simulink model "baloncuk_rov"  (R2024b)
settings: Solver=FixedStepDiscrete  StartTime=0.0  StopTime=inf  FixedStep=1e-3  RelTol=1e-3
model workspace (MAT data in the model file):
  ROTATE_CCW = 2
  ROTATE_CW = 1
  ROTATE_NONE = 0
libraries: simulink x19, utility x11, stm32f4xxblockslib x8, embeddedblockslib x2, stm32blockslib x2, dspstat3 x1
settings Model: STM32="{\"DigitalPortWrite\":[{\"ID\":\"untitled:3\"},{\"ID\":\"bldc_test:55\"},{\"ID\":\"baloncuk_rov:721\"},{\"ID\":\"baloncuk_rov:1493\"}],\"PWMOutput\":[{\"ID\":\"bldc_test:26\"},{\"ID\":\"bldc_test:37\"},{\"ID\":\"bldc_test:40\"},{\"ID\":\"bldc_test:45\"},{\"ID\":\"bldc_test:29\"},{\"ID\":\"bldc_test:74\"},{\"ID\":\"bldc_test:75\"},{\"ID\":\"bldc_test:76\"},{\"ID\":\"bldc_test:77\"},{\"ID\":\"baloncuk_rov:110\"},{\"ID\":\"baloncuk_rov:144\"},{\"ID\":\"baloncuk_rov:152\"},{\"ID\":\"baloncuk_rov:1586\"},{\"ID\":\"baloncuk_rov:1592\"}],\"TcpSend\":{\"ID\":\"bldc_test:62\"},\"TcpReceive\":{\"ID\":\"bldc_test:100\"},\"UdpReceive\":{\"ID\":\"baloncuk_rov:734\"},\"AnalogInput\":{\"ID\":\"baloncuk_rov:617\"},\"UdpSend\":{\"ID\":\"baloncuk_rov:1467\"}}"  SnapshotInterval=1000  Creator=loq  LastModifiedBy=loq
settings SolverCC: PositivePriorityOrder=on
settings OptimizationCC: UseDivisionForNetSlopeComputation=on  GainParamInheritBuiltInType=on  UseFloatMulNetSlope=on  UseSpecifiedMinMax=on  PassReuseOutputArgsAs=Individual arguments  ZeroExternalMemoryAtStartup=off  ZeroInternalMemoryAtStartup=off  NoFixptDivByZeroProtection=on  EfficientFloat2IntCast=on  LifeSpan=1  MaxStackSize=512  OptimizeBlockOrder=speed  DifferentSizesBufferReuse=on  EfficientTunableParamExpr=on
settings DebuggingCC: SignalInfNanChecking=warning  IntegerOverflowMsg=error  ParameterTunabilityLossMsg=error  AssertControl=DisableAll  SFUndirectedBroadcastEventsDiag=error
settings HardwareCC: ProdBitPerPointer=32  ProdBitPerSizeT=32  ProdBitPerPtrDiffT=32  ProdLargestAtomicInteger=Long  ProdLargestAtomicFloat=Double  ProdWordSize=32  ProdLongLongMode=on  ProdHWDeviceType=ARM Compatible->ARM Cortex-M
settings SFSimCC: SimCustomHeaderCode="#include \"bno08x_rvc_usart2_hal.h\""  SimUserSources=bno08x_rvc_usart2_hal.c  SimUserIncludeDirs=.\Core\Inc .\Core\Src .\baloncuk_rov_ert_rtw .\Drivers\CMSIS\Include .\Drivers\CMSIS\Device\ST\STM32F4xx\Include .\Drivers\STM32F4xx_HAL_Driver\Inc .\Drivers\STM32F4xx_HAL_Driver\Src  SimUserDefines=STM32F439xx  CompileTimeRecursionLimit=0  EnableRuntimeRecursion=off  MATLABDynamicMemAlloc=off
settings RTWCC: Description=Embedded Coder  SystemTargetFile=ert.tlc  HardwareBoard=STM32F4xx Based  TLCOptions="-aInlineSetEventsForThisBaseRateFcn=TLC_FALSE -aSuppressMultiTaskScheduler=TLC_FALSE   -aRateBasedStepFcn=1"  TemplateMakefile=ert_default_tmf  RTWUseSimCustomCode=on  CustomHeaderCode="#include \"bno08x_rvc_usart2_hal.h\""  CustomInclude=.\Core\Inc .\Core\Src .\baloncuk_rov_ert_rtw .\Drivers\CMSIS\Include .\Drivers\CMSIS\Device\ST\STM32F4xx\Include .\Drivers\STM32F4xx_HAL_Driver\Inc .\Drivers\STM32F4xx_HAL_Driver\Src  CustomSource=bno08x_rvc_usart2_hal.c  CustomDefine=STM32F439xx  Toolchain=GNU Tools for ARM Embedded Processors  BuildConfiguration=Faster Runs
settings CodeAppCC: ForceParamTrailComments=on  IgnoreCustomStorageClasses=off  OperatorAnnotations=on  SimulinkDataObjDesc=on  SFDataObjDesc=on  MATLABFcnDesc=on  InsertBlockDesc=on
settings ERTTargetCC: TargetLangStandard=C99 (ISO)  CodeReplacementLibrary=ARM Cortex-M  UtilityFuncGeneration=Shared location  CombineSignalStateStructs=on  SuppressErrorStatus=on  SupportNonFinite=off  ParenthesesLevel=Standards  CastingMode=Standards  GenerateSharedConstants=off  ExtModeTransport=3  ExtModeStaticAlloc=on  ExtModeStaticAllocSize=2048  ExtModeMexFile=ext_xcp  ExtModeIntrfLevel=Level2 - Open  InlinedParameterPlacement=Hierarchical  EnableSignedLeftShifts=off  EnableSignedRightShifts=off

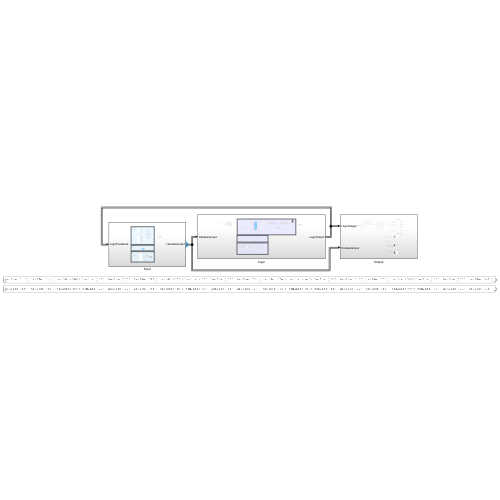
[thumbnail: Simulink's stored preview of the top-level diagram]
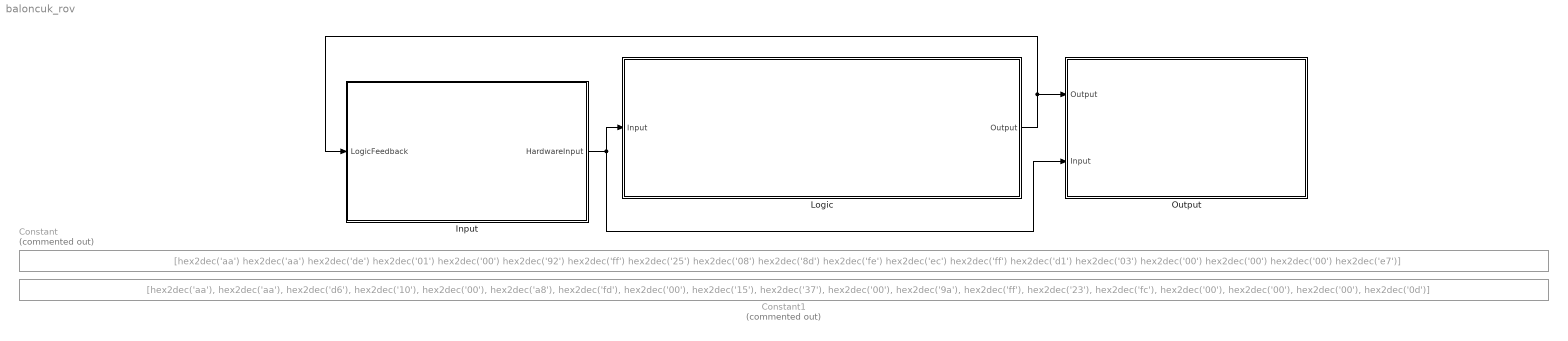
== system baloncuk_rov ==
  Constant : Constant  Commented=on  Value=[hex2dec('aa') hex2dec('aa') hex2dec('de') hex2dec('01') hex2dec('00') hex2dec('92') hex2dec('ff') hex2dec('25') hex2dec('08') hex2dec('8d') hex2dec('fe') hex2dec('ec') hex2dec('ff') hex2dec('d1') hex2dec('03') hex2dec('00') hex2dec('00') hex2dec('00') hex2dec('e7')]  OutDataTypeStr=uint8
  Constant1 : Constant  Commented=on  Value=[hex2dec('aa'), hex2dec('aa'), hex2dec('d6'), hex2dec('10'), hex2dec('00'), hex2dec('a8'), hex2dec('fd'), hex2dec('00'), hex2dec('15'), hex2dec('37'), hex2dec('00'), hex2dec('9a'), hex2dec('ff'), hex2dec('23'), hex2dec('fc'), hex2dec('00'), hex2dec('00'), hex2dec('00'), hex2dec('0d')]  OutDataTypeStr=uint8
  Input : Subsystem
  Logic : Subsystem
  Output : Subsystem
  wires:
  Input/1(HardwareInput) -> Logic/1(Input), Output/2(Input)
  Logic/1(Output) -> Input/1(LogicFeedback), Output/1(Output)

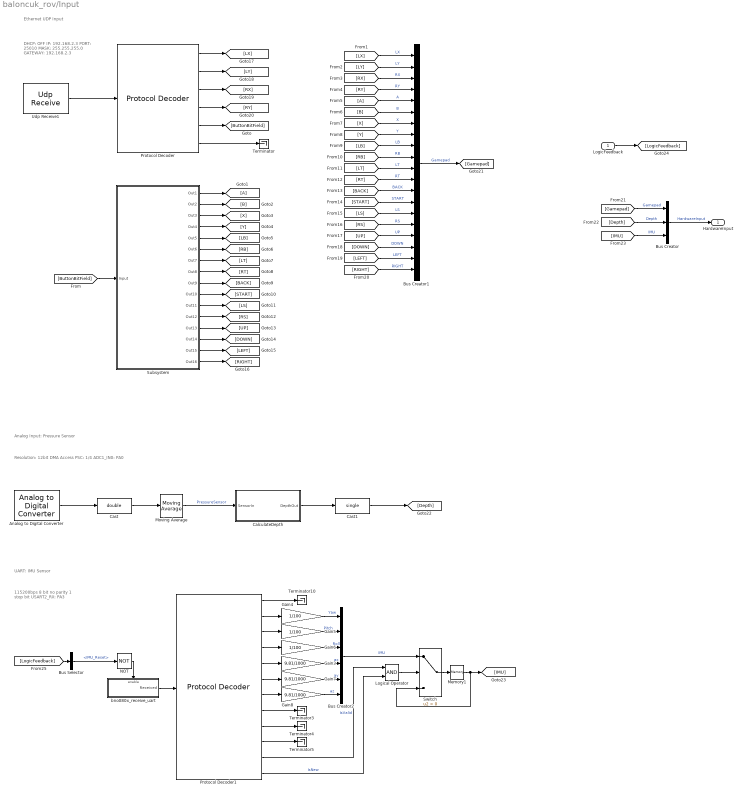
== system baloncuk_rov/Input ==
  note: Ethernet UDP Input
  note: DHCP: OFF
      | IP: 192.168.2.3
      | PORT: 25010
      | MASK: 255.255.255.0
      | GATEWAY: 192.168.2.3
  note: Analog Input: Pressure Sensor
  note: Resolution: 12bit
      | DMA Access
      | PSC: 1/4
      | ADC1_IN0: PA0
  note: UART: IMU Sensor
  note: 115200bps
      | 8 bit
      | no parity
      | 1 stop bit
      |
      | USART2_RX: PA3
  LogicFeedback : Inport
  Analog to Digital Converter : stm32f4xxblockslib/Analog to Digital Converter  ADCModule=ADC1  ConversionGroup=Regular  TriggerMode=Trigger and read  NumberOfConversions=1  EnableBufferConv=off  BufferLength=1  OutputStatus=off  SampleTime=-1  EnableSimPort=off  hoistedMaskSrc=ECSoC/ECSimCodegen/Analog to Digital Converter
  Bus Creator : BusCreator  Inputs=3
  Bus Creator1 : BusCreator  Inputs=20
  Bus Creator2 : BusCreator  Inputs=6
  Bus Selector : BusSelector  OutputSignals=IMU_Bus.IMU_Reset
  CalculateDepth : Subsystem
  Cast : DataTypeConversion  OutDataTypeStr=double  SaturateOnIntegerOverflow=off  RndMeth=Floor
  Cast1 : DataTypeConversion  OutDataTypeStr=single  SaturateOnIntegerOverflow=off  RndMeth=Floor
  From5 : From
  Gain3 : Gain  Gain=9.81/1000  OutDataTypeStr=single
  Gain4 : Gain  Gain=1/100  OutDataTypeStr=single
  Gain5 : Gain  Gain=1/100  OutDataTypeStr=single
  Gain6 : Gain  Gain=1/100  OutDataTypeStr=single
  Gain7 : Gain  Gain=9.81/1000  OutDataTypeStr=single
  Gain8 : Gain  Gain=9.81/1000  OutDataTypeStr=single
  Goto1 : Goto
  Logical Operator : Logic  AllPortsSameDT=off  OutDataTypeStr=boolean
  Memory1 : Memory
  Moving Average : dspstat3/Moving Average  Method=Sliding window  ForgettingFactorPort=off  SpecifyWindowLength=on  WindowLength=1/0.005  OverlapLength=199  AllowArbitraryInputLength=off  ForgettingFactor=0.9  SimulateUsing=Interpreted execution
  NOT : Logic  Operator=NOT  IconShape=distinctive  AllPortsSameDT=off  OutDataTypeStr=boolean
  Protocol Decoder : embeddedblockslib/Protocol Decoder  IsParseCSV=off  Header=[13]  FieldTable={ 'LX', '1', 'int8', 'Little endian'; 'LY', '1', 'int8', 'Little endian'; 'RX', '1', 'int8', 'Little endian'; 'RY', '1', 'int8', 'Little endian'; 'ButtonBitField', '1', 'uint16', 'Little endian' }  IsVariableSizeLastField=off  MaxVariableSizeFieldLength=[]  IsChecksumRequired=off  ChecksumAlgorithm=XOR of bytes  ChecksumSize=[]  TerminatorOption=Custom terminator  CustomTerminatorVal=[10]  IsInputLengthAvailable=off
      settings: LibrarySourceBlock=stmutilitieslib/Protocol Decoder
  Protocol Decoder1 : embeddedblockslib/Protocol Decoder  IsParseCSV=off  Header=[hex2dec('aa') hex2dec('aa')]  FieldTable={ 'Index', '1', 'uint8', 'Little endian'; 'Yaw', '1', 'int16', 'Little endian'; 'Pitch', '1', 'int16', 'Little endian'; 'Roll', '1', 'int16', 'Little endian'; 'X_Accel', '1', 'int16', 'Little endian'; 'Y_Accel', '1', 'int16', 'Little endian'; 'Z_Accel', '1', 'int16', 'Little endian'; 'Res_0', '1', 'uint8', 'Little endian'; 'Res_1', '1', 'uint8', 'Little endian'; 'Res_2', '1', 'uint8', 'Little endian' }  IsVariableSizeLastField=off  MaxVariableSizeFieldLength=[]  IsChecksumRequired=on  ChecksumAlgorithm=Custom algorithm  ChecksumSize=1  ChecksumFilepath=C:\Users\loq\Documents\MATLAB\baloncuk_rov\bno08x_checksum.m  TerminatorOption=<none>  CustomTerminatorVal=[10]  IsInputLengthAvailable=off
      settings: LibrarySourceBlock=stmutilitieslib/Protocol Decoder
  Subsystem : Subsystem
  Switch : Switch  Criteria=u2 > Threshold  SaturateOnIntegerOverflow=off  InputSameDT=off
  Terminator{,3..5,10} (5 alike) : Terminator
  Udp Receive1 : stm32blockslib/Udp Receive  Direction=Receive  RemoteIPAddress=192.168.2.2  LocalPort=25010  RemoteIPPort=25002  ByteOrder=LittleEndian  BlockingMode=off  BlockTimeout=0.1  DataType=uint8  DataLength=8  OutputStatus=off  SampleTime=-1
      settings: LibrarySourceBlock=stm32f4xxblockslib/Udp Receive
  bno080x_receive_uart : Subsystem  TreatAsAtomicUnit=on
  HardwareInput : Outport
  wires:
  Subsystem/15(Out15) -> [LEFT]
  [ButtonBitField] -> Subsystem/1(Input)
  Subsystem/12(Out12) -> [RS]
  Subsystem/14(Out14) -> [DOWN]
  Subsystem/1(Out1) -> Goto1/1
  Protocol Decoder/6 -> Terminator/1
  Protocol Decoder/2 -> [LY]
  Subsystem/3(Out3) -> [X]
  Protocol Decoder/4 -> [RY]
  Subsystem/10(Out10) -> [START]
  Subsystem/11(Out11) -> [LS]
  Subsystem/7(Out7) -> [LT]
  Protocol Decoder/5 -> [ButtonBitField]
  Subsystem/6(Out6) -> [RB]
  Subsystem/8(Out8) -> [RT]
  Udp Receive1/1 -> Protocol Decoder/1
  Protocol Decoder/1 -> [LX]
  Subsystem/5(Out5) -> [LB]
  Protocol Decoder/3 -> [RX]
  Subsystem/16(Out16) -> [RIGHT]
  Subsystem/2(Out2) -> [B]
  Subsystem/9(Out9) -> [BACK]
  Subsystem/4(Out4) -> [Y]
  Subsystem/13(Out13) -> [UP]
  [LX] -> Bus Creator1/1  "LX"
  [LY] -> Bus Creator1/2  "LY"
  [RX] -> Bus Creator1/3  "RX"
  [RY] -> Bus Creator1/4  "RY"
  From5/1 -> Bus Creator1/5  "A"
  [B] -> Bus Creator1/6  "B"
  [X] -> Bus Creator1/7  "X"
  [Y] -> Bus Creator1/8  "Y"
  [LB] -> Bus Creator1/9  "LB"
  [RB] -> Bus Creator1/10  "RB"
  [LT] -> Bus Creator1/11  "LT"
  [RT] -> Bus Creator1/12  "RT"
  [BACK] -> Bus Creator1/13  "BACK"
  [START] -> Bus Creator1/14  "START"
  [LS] -> Bus Creator1/15  "LS"
  [RS] -> Bus Creator1/16  "RS"
  [UP] -> Bus Creator1/17  "UP"
  [DOWN] -> Bus Creator1/18  "DOWN"
  [LEFT] -> Bus Creator1/19  "LEFT"
  [RIGHT] -> Bus Creator1/20  "RIGHT"
  Bus Creator/1 -> HardwareInput/1  "HardwareInput"
  Bus Creator1/1 -> [Gamepad]  "Gamepad"
  [Gamepad] -> Bus Creator/1  "Gamepad"
  Cast/1 -> Moving Average/1
  Analog to Digital Converter/1 -> Cast/1
  Moving Average/1 -> CalculateDepth/1(SensorIn)  "PressureSensor"
  CalculateDepth/1(DepthOut) -> Cast1/1
  [Depth] -> Bus Creator/2  "Depth"
  [IMU] -> Bus Creator/3  "IMU"
  Gain3/1 -> Bus Creator2/4  "ax"
  Protocol Decoder1/6 -> Gain7/1
  Protocol Decoder1/5 -> Gain3/1
  Gain7/1 -> Bus Creator2/5  "ay"
  Bus Creator2/1 -> Switch/1  "IMU"
  Protocol Decoder1/1 -> Terminator10/1
  Gain6/1 -> Bus Creator2/3  "Roll"
  Protocol Decoder1/4 -> Gain6/1
  Protocol Decoder1/2 -> Gain4/1
  Gain4/1 -> Bus Creator2/1  "Yaw"
  Protocol Decoder1/9 -> Terminator4/1
  Gain8/1 -> Bus Creator2/6  "az"
  Protocol Decoder1/12 -> Logical Operator/2  "IsNew"
  Protocol Decoder1/7 -> Gain8/1
  Protocol Decoder1/11 -> Logical Operator/1  "IsValid"
  Protocol Decoder1/8 -> Terminator3/1
  Gain5/1 -> Bus Creator2/2  "Pitch"
  Protocol Decoder1/3 -> Gain5/1
  Protocol Decoder1/10 -> Terminator5/1
  Logical Operator/1 -> Switch/2
  Switch/1 -> Memory1/1
  Memory1/1 -> Switch/3, [IMU]
  bno080x_receive_uart/1(Received) -> Protocol Decoder1/1
  NOT/1 -> bno080x_receive_uart/Enable
  LogicFeedback/1 -> [LogicFeedback]
  [LogicFeedback] -> Bus Selector/1
  Bus Selector/1 -> NOT/1  "<IMU_Reset>"
  Cast1/1 -> [Depth]

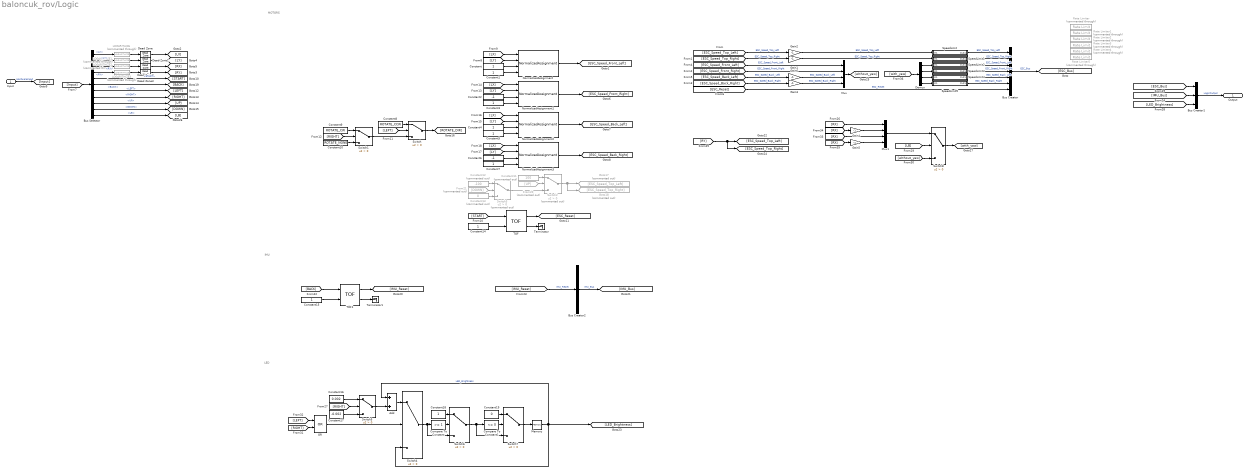
== system baloncuk_rov/Logic ==
  note: LED
  note: MOTORS
  note: IMU
  Input : Inport
  Add : Sum
  Bus Creator : BusCreator  Inputs=7
  Bus Creator1 : BusCreator  Inputs=3
  Bus Creator2 : BusCreator  Inputs=1
  Bus Selector : BusSelector  OutputSignals=Gamepad.LX,Gamepad.LY,Gamepad.RX,Gamepad.RY,Gamepad.START,Gamepad.BACK,Gamepad.LEFT,Gamepad.RIGHT,Gamepad.UP,Gamepad.DOWN,Gamepad.LB
  Compare To Constant : simulink/Logic and Bit Operations/Compare To Constant  relop=>=  const=1  OutDataTypeStr=boolean
  Compare To Constant1 : simulink/Logic and Bit Operations/Compare To Constant  relop=<=  const=0  OutDataTypeStr=boolean
  Constant{,1,3..5,7} (6 alike) : Constant  OutDataTypeStr=int8
  Constant10 : Constant  Value=ROTATE_NONE
  Constant11 : Constant  Commented=on  Value=100  OutDataTypeStr=int8
  Constant12 : Constant  Commented=on  Value=-100  OutDataTypeStr=int8
  Constant13 : Constant  Commented=on  Value=0  OutDataTypeStr=int8
  Constant14 : Constant  OutDataTypeStr=single
  Constant15 : Constant  OutDataTypeStr=single
  Constant16 : Constant  Value=0.002
  Constant17 : Constant  Value=-0.002
  Constant18 : Constant
  Constant19 : Constant  Value=0
  Constant2 : Constant  Value=-1  OutDataTypeStr=int8
  Constant6 : Constant  Value=-1  OutDataTypeStr=int8
  Constant8 : Constant  Value=ROTATE_CCW
  Constant9 : Constant  Value=ROTATE_CW
  Dead Zone{,1..3} (4 alike) : DeadZone  LowerValue=-5  UpperValue=5
  Demux : Demux
  From20 : From  Commented=on  GotoTag=UP
  From21 : From  Commented=on  GotoTag=DOWN
  Gain{1..4,6} (5 alike) : Gain  Gain=-1  OutDataTypeStr=int8
  Gain5 : Gain  Gain=-1  ParamDataTypeStr=int8  OutDataTypeStr=int8
  Goto17 : Goto  Commented=on  GotoTag=ESC_Speed_Top_Left
  Goto18 : Goto  Commented=on  GotoTag=ESC_Speed_Top_Right
  LOGARITHIZE{,1..3} (4 alike) : utility/LOGARITHIZE  Commented=through  SystemSampleTime=-1  VariantActivationTime=update diagram  AllowFlexibleInterface=on  Latency=0  AutoFrameSizeCalculation=off
  Memory : Memory  InitialCondition=0.00  InheritSampleTime=on
  Mux : Mux
  Mux1 : Mux
  NormalizedAssignment{,1..3} (4 alike) : utility/NormalizedAssignment  SystemSampleTime=-1  VariantActivationTime=update diagram  AllowFlexibleInterface=on  Latency=0  AutoFrameSizeCalculation=off
  OR : Logic  Operator=OR  AllPortsSameDT=off  OutDataTypeStr=boolean
  Rate Limiter{,1..5} (6 alike) : RateLimiter  Commented=through  RisingSlewLimit=10  FallingSlewLimit=-10  SampleTimeMode=inherited
  SpeedLimit : Subsystem
  SpeedLimit1 : Subsystem
  SpeedLimit2 : Subsystem
  SpeedLimit3 : Subsystem
  SpeedLimit4 : Subsystem
  SpeedLimit5 : Subsystem
  Switch{,1,4..8} (7 alike) : Switch  Criteria=u2 > Threshold  SaturateOnIntegerOverflow=off  InputSameDT=off
  Switch2 : Switch  Commented=on  Criteria=u2 > Threshold  SaturateOnIntegerOverflow=off  InputSameDT=off
  Switch3 : Switch  Commented=on  Criteria=u2 > Threshold  SaturateOnIntegerOverflow=off  InputSameDT=off
  TOF : utility/TOF  SystemSampleTime=-1  VariantActivationTime=update diagram  AllowFlexibleInterface=on  Latency=0  AutoFrameSizeCalculation=off
  TOF1 : utility/TOF  SystemSampleTime=-1  VariantActivationTime=update diagram  AllowFlexibleInterface=on  Latency=0  AutoFrameSizeCalculation=off
  Terminator : Terminator
  Terminator1 : Terminator
  Output : Outport
  wires:
  [ESC_Speed_Top_Left] -> Gain2/1  "ESC_Speed_Top_Left"
  [ESC_Speed_Top_Right] -> Gain1/1  "ESC_Speed_Top_Right"
  [ESC_Speed_Front_Right] -> Mux/2  "ESC_Speed_Front_Right"
  [ESC_Speed_Back_Left] -> Gain6/1  "ESC_Speed_Back_Left"
  [ESC_Speed_Front_Left] -> Mux/1  "ESC_Speed_Front_Left"
  [ESC_Reset] -> Bus Creator/7  "ESC_Reset"
  Bus Creator/1 -> [ESC_Bus]  "ESC_Bus"
  Input/1 -> [Input]  "HardwareInput"
  Bus Selector/1 -> LOGARITHIZE/1  "<LX>"
  Bus Selector/4 -> LOGARITHIZE3/1  "<RY>"
  Bus Selector/2 -> LOGARITHIZE1/1  "<LY>"
  Bus Selector/3 -> LOGARITHIZE2/1  "<RX>"
  NormalizedAssignment/1 -> [ESC_Speed_Front_Left]
  [LX] -> NormalizedAssignment/1
  [LY] -> NormalizedAssignment/2
  Constant/1 -> NormalizedAssignment/3
  Constant1/1 -> NormalizedAssignment/4
  Constant3/1 -> NormalizedAssignment1/4
  Constant2/1 -> NormalizedAssignment1/3
  [LY] -> NormalizedAssignment1/2
  [LX] -> NormalizedAssignment1/1
  NormalizedAssignment1/1 -> [ESC_Speed_Front_Right]
  NormalizedAssignment2/1 -> [ESC_Speed_Back_Left]
  [LX] -> NormalizedAssignment2/1
  [LY] -> NormalizedAssignment2/2
  Constant4/1 -> NormalizedAssignment2/3
  Constant5/1 -> NormalizedAssignment2/4
  Constant7/1 -> NormalizedAssignment3/4
  Constant6/1 -> NormalizedAssignment3/3
  [LX] -> NormalizedAssignment3/1
  NormalizedAssignment3/1 -> [ESC_Speed_Back_Right]
  [Input] -> Bus Selector/1
  Bus Selector/5 -> [START]  "<START>"
  Bus Selector/7 -> [LEFT]  "<LEFT>"
  Bus Selector/8 -> [RIGHT]  "<RIGHT>"
  Bus Selector/9 -> [UP]  "<UP>"
  Bus Selector/10 -> [DOWN]  "<DOWN>"
  [LEFT] -> Switch/2
  Constant8/1 -> Switch/1
  Constant9/1 -> Switch1/1
  [RIGHT] -> Switch1/2
  Switch1/1 -> Switch/3
  Switch/1 -> [ROTATE_DIR]
  Constant10/1 -> Switch1/3
  [ESC_Bus] -> Bus Creator1/1
  Bus Creator1/1 -> Output/1  "LogicOutput"
  Switch2/1 -> Goto18/1, Goto17/1
  From20/1 -> Switch2/2
  Constant11/1 -> Switch2/1
  Constant12/1 -> Switch3/1
  From21/1 -> Switch3/2
  Switch3/1 -> Switch2/3
  Constant13/1 -> Switch3/3
  [START] -> TOF/1
  TOF/1 -> [ESC_Reset]
  Constant14/1 -> TOF/2
  TOF/2 -> Terminator/1
  LOGARITHIZE/1 -> Dead Zone/1
  LOGARITHIZE1/1 -> Dead Zone1/1
  LOGARITHIZE2/1 -> Dead Zone2/1
  LOGARITHIZE3/1 -> Dead Zone3/1
  Bus Selector/6 -> [BACK]  "<BACK>"
  TOF1/2 -> Terminator1/1
  Constant15/1 -> TOF1/2
  TOF1/1 -> [IMU_Reset]
  [BACK] -> TOF1/1
  Bus Creator2/1 -> [IMU_Bus]  "IMU_Bus"
  [IMU_Reset] -> Bus Creator2/1  "IMU_Reset"
  [IMU_Bus] -> Bus Creator1/2
  [LED_Brightness] -> Bus Creator1/3
  Switch4/1 -> Switch6/3, Compare To Constant/1
  [LEFT] -> OR/1
  Switch7/1 -> Memory/1
  Constant17/1 -> Switch5/3
  [RIGHT] -> OR/2
  Constant16/1 -> Switch5/1
  Switch5/1 -> Add/2
  Memory/1 -> [LED_Brightness], Add/1, Switch4/3  "LED_Brightness"
  [RIGHT] -> Switch5/2
  OR/1 -> Switch4/2
  Constant18/1 -> Switch6/1
  Constant19/1 -> Switch7/1
  Compare To Constant1/1 -> Switch7/2
  Add/1 -> Switch4/1
  Switch6/1 -> Switch7/3, Compare To Constant1/1
  Compare To Constant/1 -> Switch6/2
  Gain1/1 -> SpeedLimit1/1(In1)  "ESC_Speed_Top_Right"
  [LY] -> NormalizedAssignment3/2
  Dead Zone/1 -> [LX]
  Dead Zone1/1 -> [LY]
  Dead Zone2/1 -> [RX]
  Dead Zone3/1 -> [RY]
  SpeedLimit/1(Out1) -> Bus Creator/1  "ESC_Speed_Top_Left"
  SpeedLimit1/1(Out1) -> Bus Creator/2  "ESC_Speed_Top_Right"
  SpeedLimit2/1(Out1) -> Bus Creator/3  "ESC_Speed_Front_Left"
  SpeedLimit3/1(Out1) -> Bus Creator/4  "ESC_Speed_Front_Right"
  SpeedLimit4/1(Out1) -> Bus Creator/5  "ESC_Speed_Back_Left"
  SpeedLimit5/1(Out1) -> Bus Creator/6  "ESC_Speed_Back_Right"
  [RY] -> [ESC_Speed_Top_Right], [ESC_Speed_Top_Left]
  [ESC_Speed_Back_Right] -> Gain3/1  "ESC_Speed_Back_Right"
  Mux/1 -> [without_yaw]
  Bus Selector/11 -> [LB]  "<LB>"
  [LB] -> Switch8/2
  [without_yaw] -> Switch8/3
  [RX] -> Mux1/1
  [RX] -> Mux1/3
  [RX] -> Gain4/1
  [RX] -> Gain5/1
  Gain4/1 -> Mux1/2
  Gain5/1 -> Mux1/4
  Mux1/1 -> Switch8/1
  Switch8/1 -> [with_yaw]
  [with_yaw] -> Demux/1
  Demux/1 -> SpeedLimit2/1(In1)
  Demux/2 -> SpeedLimit3/1(In1)
  Demux/3 -> SpeedLimit4/1(In1)
  Demux/4 -> SpeedLimit5/1(In1)
  Gain2/1 -> SpeedLimit/1(In1)  "ESC_Speed_Top_Left"
  Gain3/1 -> Mux/4  "ESC_Speed_Back_Right"
  Gain6/1 -> Mux/3  "ESC_Speed_Back_Left"

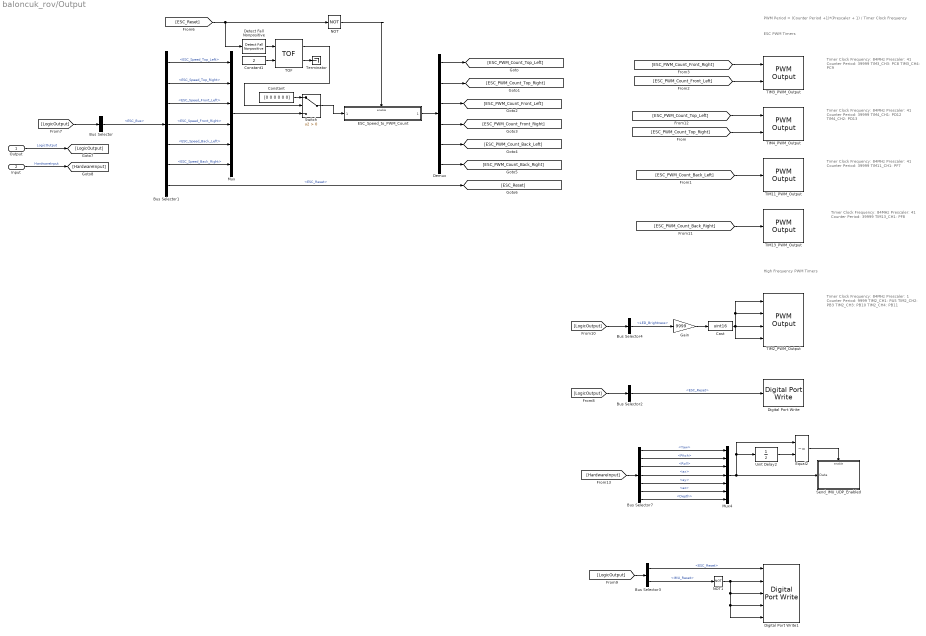
== system baloncuk_rov/Output ==
  note: PWM Period = (Counter Period +1)*(Prescaler + 1) / Timer Clock Frequency
  note: ESC PWM Timers
  note: Timer Clock Frequency: 84MHz
      | Prescaler: 41
      | Counter Period: 39999
      |
      | TIM3_CH3: PC8
      | TIM3_CH4: PC9
  note: High Frequency PWM Timers
  note: Timer Clock Frequency: 84MHz
      | Prescaler: 1
      | Counter Period: 9999
      |
      | TIM2_CH1: PA5
      | TIM2_CH2: PB3
      | TIM2_CH3: PB10
      | TIM2_CH4: PB11
  note: Timer Clock Frequency: 84MHz
      | Prescaler: 41
      | Counter Period: 39999
      |
      | TIM4_CH1: PD12
      | TIM4_CH2: PD13
  note: Timer Clock Frequency: 84MHz
      | Prescaler: 41
      | Counter Period: 39999
      |
      | TIM11_CH1: PF7
  note: Timer Clock Frequency: 84MHz
      | Prescaler: 41
      | Counter Period: 39999
      |
      | TIM13_CH1: PF8
  Output : Inport
  Input : Inport  Port=2
  Bus Selector : BusSelector  OutputSignals=ESC_Bus
  Bus Selector1 : BusSelector  OutputSignals=ESC_Speed_Top_Left,ESC_Speed_Top_Right,ESC_Speed_Front_Left,ESC_Speed_Front_Right,ESC_Speed_Back_Left,ESC_Speed_Back_Right,ESC_Reset
  Bus Selector2 : BusSelector  OutputSignals=ESC_Bus.ESC_Reset
  Bus Selector3 : BusSelector  OutputSignals=ESC_Bus.ESC_Reset,IMU_Bus.IMU_Reset
  Bus Selector4 : BusSelector  OutputSignals=LED_Brightness
  Bus Selector7 : BusSelector  OutputSignals=IMU.Yaw,IMU.Pitch,IMU.Roll,IMU.ax,IMU.ay,IMU.az,Depth
  Cast : DataTypeConversion  OutDataTypeStr=uint16  SaturateOnIntegerOverflow=off  RndMeth=Floor
  Constant : Constant  Value=[0 0 0 0 0 0]
  Constant1 : Constant  Value=2  OutDataTypeStr=single
  Demux : Demux  Outputs=6
  Detect Fall Nonpositive : simulink/Logic and Bit Operations/Detect Fall Nonpositive  vinit=0  OutDataTypeStr=boolean
  Digital Port Write : stm32f4xxblockslib/Digital Port Write  PortName=GPIOB  PinNumber=7  ReadOperation=off  IOAsArray=off  EnableSimPort=off  hoistedMaskSrc=ECSoC/ECSimCodegen/Digital Port Write
  Digital Port Write1 : stm32f4xxblockslib/Digital Port Write  PortName=GPIOE  PinNumber=[2 3 4 5 6]  ReadOperation=off  IOAsArray=off  EnableSimPort=off  hoistedMaskSrc=ECSoC/ECSimCodegen/Digital Port Write
  ESC_Speed_to_PWM_Count : Subsystem  ReferencedSubsystem=ESC_Speed_to_PWM_Count
  Equal2 : RelationalOperator  Operator=~=  OutDataTypeStr=boolean  RndMeth=Simplest  InputSameDT=off
  Gain : Gain  Gain=9999
  Mux : Mux  Inputs=6
  Mux4 : Mux  Inputs=7
  NOT : Logic  Operator=NOT  IconShape=distinctive  AllPortsSameDT=off  OutDataTypeStr=boolean
  NOT1 : Logic  Operator=NOT  IconShape=distinctive  AllPortsSameDT=off  OutDataTypeStr=boolean
  Send_IMU_UDP_Enabled : Subsystem  TreatAsAtomicUnit=on
  Switch : Switch  Criteria=u2 > Threshold  SaturateOnIntegerOverflow=off  InputSameDT=off
  TIM11_PWM_Output : stm32f4xxblockslib/PWM Output  TimerModule=TIM11  DutycycleUnits=Counts  EnableChannel1=on  EnableChannel2=on  EnableChannel3=on  EnableChannel4=on  EnableCounterInput=off  EnableMainOutputInput=off  EnableFrequencyInput=off  SetRCAfterCE=off  OutputDirection=off  OutputMainOutputEnableStatus=off  SampleTime=0.1  EnableSimPort=off  EnableUpdateEvent=off  EnableCaptureCompare1Event=off  EnableCaptureCompare2Event=off  EnableCaptureCompare3Event=off  EnableCaptureCompare4Event=off  EnableTriggerEvent=off  EnableBreakEvent=off  ProcessorFamily=STM32F4  hoistedMaskSrc=ECSoC/ECSimCodegen/PWM Output
  TIM13_PWM_Output : stm32f4xxblockslib/PWM Output  TimerModule=TIM13  DutycycleUnits=Counts  EnableChannel1=on  EnableChannel2=on  EnableChannel3=on  EnableChannel4=on  EnableCounterInput=off  EnableMainOutputInput=off  EnableFrequencyInput=off  SetRCAfterCE=off  OutputDirection=off  OutputMainOutputEnableStatus=off  SampleTime=0.1  EnableSimPort=off  EnableUpdateEvent=off  EnableCaptureCompare1Event=off  EnableCaptureCompare2Event=off  EnableCaptureCompare3Event=off  EnableCaptureCompare4Event=off  EnableTriggerEvent=off  EnableBreakEvent=off  ProcessorFamily=STM32F4  hoistedMaskSrc=ECSoC/ECSimCodegen/PWM Output
  TIM2_PWM_Output : stm32f4xxblockslib/PWM Output  TimerModule=TIM2  DutycycleUnits=Counts  EnableChannel1=on  EnableChannel2=on  EnableChannel3=on  EnableChannel4=on  EnableCounterInput=off  EnableMainOutputInput=off  EnableFrequencyInput=off  SetRCAfterCE=off  OutputDirection=off  OutputMainOutputEnableStatus=off  SampleTime=0.1  EnableSimPort=off  EnableUpdateEvent=off  EnableCaptureCompare1Event=off  EnableCaptureCompare2Event=off  EnableCaptureCompare3Event=off  EnableCaptureCompare4Event=off  EnableTriggerEvent=off  EnableBreakEvent=off  ProcessorFamily=STM32F4  hoistedMaskSrc=ECSoC/ECSimCodegen/PWM Output
  TIM3_PWM_Output : stm32f4xxblockslib/PWM Output  TimerModule=TIM3  DutycycleUnits=Counts  EnableChannel1=off  EnableChannel2=off  EnableChannel3=on  EnableChannel4=on  EnableCounterInput=off  EnableMainOutputInput=off  EnableFrequencyInput=off  SetRCAfterCE=off  OutputDirection=off  OutputMainOutputEnableStatus=off  SampleTime=0.1  EnableSimPort=off  EnableUpdateEvent=off  EnableCaptureCompare1Event=off  EnableCaptureCompare2Event=off  EnableCaptureCompare3Event=off  EnableCaptureCompare4Event=off  EnableTriggerEvent=off  EnableBreakEvent=off  ProcessorFamily=STM32F4  hoistedMaskSrc=ECSoC/ECSimCodegen/PWM Output
  TIM4_PWM_Output : stm32f4xxblockslib/PWM Output  TimerModule=TIM4  DutycycleUnits=Counts  EnableChannel1=on  EnableChannel2=on  EnableChannel3=off  EnableChannel4=off  EnableCounterInput=off  EnableMainOutputInput=off  EnableFrequencyInput=off  SetRCAfterCE=off  OutputDirection=off  OutputMainOutputEnableStatus=off  SampleTime=0.1  EnableSimPort=off  EnableUpdateEvent=off  EnableCaptureCompare1Event=off  EnableCaptureCompare2Event=off  EnableCaptureCompare3Event=off  EnableCaptureCompare4Event=off  EnableTriggerEvent=off  EnableBreakEvent=off  ProcessorFamily=STM32F4  hoistedMaskSrc=ECSoC/ECSimCodegen/PWM Output
  TOF : utility/TOF  SystemSampleTime=-1  VariantActivationTime=update diagram  AllowFlexibleInterface=on  Latency=0  AutoFrameSizeCalculation=off
  Terminator : Terminator
  Unit Delay2 : UnitDelay  SampleTime=-1  HasFrameUpgradeWarning=on
  wires:
  [LogicOutput] -> Bus Selector/1
  Bus Selector/1 -> Bus Selector1/1  "<ESC_Bus>"
  [ESC_PWM_Count_Top_Left] -> TIM4_PWM_Output/1
  [ESC_PWM_Count_Top_Right] -> TIM4_PWM_Output/2
  Bus Selector1/7 -> [ESC_Reset]  "<ESC_Reset>"
  Demux/1 -> [ESC_PWM_Count_Top_Left]
  Demux/2 -> [ESC_PWM_Count_Top_Right]
  Demux/3 -> [ESC_PWM_Count_Front_Left]
  Demux/4 -> [ESC_PWM_Count_Front_Right]
  Demux/5 -> [ESC_PWM_Count_Back_Left]
  Demux/6 -> [ESC_PWM_Count_Back_Right]
  [ESC_Reset] -> Detect Fall Nonpositive/1, NOT/1
  NOT/1 -> ESC_Speed_to_PWM_Count/Enable
  ESC_Speed_to_PWM_Count/1 -> Demux/1
  Output/1 -> [LogicOutput]  "LogicOutput"
  [LogicOutput] -> Bus Selector2/1
  Bus Selector1/1 -> Mux/1  "<ESC_Speed_Top_Left>"
  Bus Selector1/2 -> Mux/2  "<ESC_Speed_Top_Right>"
  Bus Selector1/3 -> Mux/3  "<ESC_Speed_Front_Left>"
  Bus Selector1/4 -> Mux/4  "<ESC_Speed_Front_Right>"
  Bus Selector1/5 -> Mux/5  "<ESC_Speed_Back_Left>"
  Bus Selector1/6 -> Mux/6  "<ESC_Speed_Back_Right>"
  Bus Selector2/1 -> Digital Port Write/1  "<ESC_Reset>"
  Mux/1 -> Switch/3
  Switch/1 -> ESC_Speed_to_PWM_Count/1
  Constant/1 -> Switch/1
  Constant1/1 -> TOF/2
  Detect Fall Nonpositive/1 -> TOF/1
  TOF/2 -> Terminator/1
  TOF/1 -> Switch/2
  Input/1 -> [HardwareInput]  "HardwareInput"
  Equal2/1 -> Send_IMU_UDP_Enabled/Enable
  [HardwareInput] -> Bus Selector7/1
  Mux4/1 -> Send_IMU_UDP_Enabled/1(Data), Unit Delay2/1, Equal2/1
  Unit Delay2/1 -> Equal2/2
  Bus Selector7/1 -> Mux4/1  "<Yaw>"
  Bus Selector7/2 -> Mux4/2  "<Pitch>"
  Bus Selector7/3 -> Mux4/3  "<Roll>"
  Bus Selector7/4 -> Mux4/4  "<ax>"
  Bus Selector7/5 -> Mux4/5  "<ay>"
  Bus Selector7/6 -> Mux4/6  "<az>"
  Bus Selector3/1 -> Digital Port Write1/1  "<ESC_Reset>"
  [LogicOutput] -> Bus Selector3/1
  Bus Selector3/2 -> NOT1/1  "<IMU_Reset>"
  NOT1/1 -> Digital Port Write1/3, Digital Port Write1/4, Digital Port Write1/5, Digital Port Write1/2
  Bus Selector4/1 -> Gain/1  "<LED_Brightness>"
  [LogicOutput] -> Bus Selector4/1
  Gain/1 -> Cast/1
  Cast/1 -> TIM2_PWM_Output/2, TIM2_PWM_Output/1, TIM2_PWM_Output/4, TIM2_PWM_Output/3
  [ESC_PWM_Count_Back_Left] -> TIM11_PWM_Output/1
  [ESC_PWM_Count_Back_Right] -> TIM13_PWM_Output/1
  Bus Selector7/7 -> Mux4/7  "<Depth>"
  [ESC_PWM_Count_Front_Left] -> TIM3_PWM_Output/2
  [ESC_PWM_Count_Front_Right] -> TIM3_PWM_Output/1

== system baloncuk_rov/Input/CalculateDepth ==
  SensorIn : Inport
  DepthOut : Outport
  wires:
  SensorIn/1 -> DepthOut/1

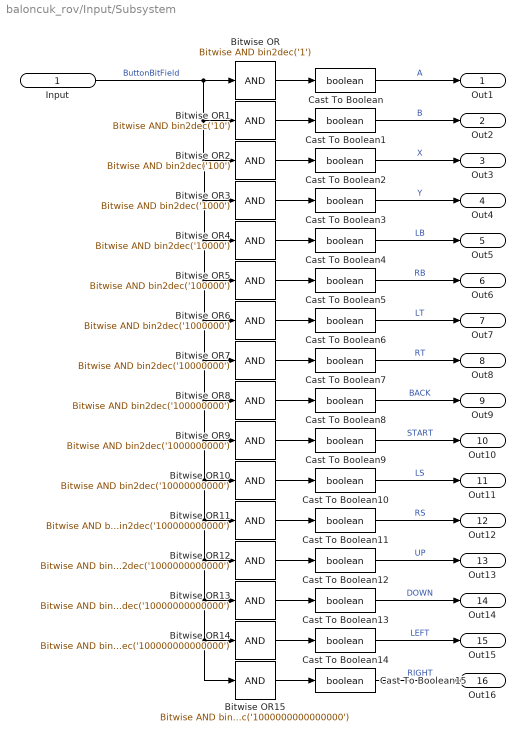
== system baloncuk_rov/Input/Subsystem ==
  Input : Inport  OutDataTypeStr=uint16
  Bitwise OR : simulink/Logic and Bit Operations/Bitwise Operator  logicop=AND  UseBitMask=on  BitMask=bin2dec('1')  BitMaskRealWorld=Stored Integer
  Bitwise OR1 : simulink/Logic and Bit Operations/Bitwise Operator  logicop=AND  UseBitMask=on  BitMask=bin2dec('10')  BitMaskRealWorld=Stored Integer
  Bitwise OR10 : simulink/Logic and Bit Operations/Bitwise Operator  logicop=AND  UseBitMask=on  BitMask=bin2dec('10000000000')  BitMaskRealWorld=Stored Integer
  Bitwise OR11 : simulink/Logic and Bit Operations/Bitwise Operator  logicop=AND  UseBitMask=on  BitMask=bin2dec('100000000000')  BitMaskRealWorld=Stored Integer
  Bitwise OR12 : simulink/Logic and Bit Operations/Bitwise Operator  logicop=AND  UseBitMask=on  BitMask=bin2dec('1000000000000')  BitMaskRealWorld=Stored Integer
  Bitwise OR13 : simulink/Logic and Bit Operations/Bitwise Operator  logicop=AND  UseBitMask=on  BitMask=bin2dec('10000000000000')  BitMaskRealWorld=Stored Integer
  Bitwise OR14 : simulink/Logic and Bit Operations/Bitwise Operator  logicop=AND  UseBitMask=on  BitMask=bin2dec('100000000000000')  BitMaskRealWorld=Stored Integer
  Bitwise OR15 : simulink/Logic and Bit Operations/Bitwise Operator  logicop=AND  UseBitMask=on  BitMask=bin2dec('1000000000000000')  BitMaskRealWorld=Stored Integer
  Bitwise OR2 : simulink/Logic and Bit Operations/Bitwise Operator  logicop=AND  UseBitMask=on  BitMask=bin2dec('100')  BitMaskRealWorld=Stored Integer
  Bitwise OR3 : simulink/Logic and Bit Operations/Bitwise Operator  logicop=AND  UseBitMask=on  BitMask=bin2dec('1000')  BitMaskRealWorld=Stored Integer
  Bitwise OR4 : simulink/Logic and Bit Operations/Bitwise Operator  logicop=AND  UseBitMask=on  BitMask=bin2dec('10000')  BitMaskRealWorld=Stored Integer
  Bitwise OR5 : simulink/Logic and Bit Operations/Bitwise Operator  logicop=AND  UseBitMask=on  BitMask=bin2dec('100000')  BitMaskRealWorld=Stored Integer
  Bitwise OR6 : simulink/Logic and Bit Operations/Bitwise Operator  logicop=AND  UseBitMask=on  BitMask=bin2dec('1000000')  BitMaskRealWorld=Stored Integer
  Bitwise OR7 : simulink/Logic and Bit Operations/Bitwise Operator  logicop=AND  UseBitMask=on  BitMask=bin2dec('10000000')  BitMaskRealWorld=Stored Integer
  Bitwise OR8 : simulink/Logic and Bit Operations/Bitwise Operator  logicop=AND  UseBitMask=on  BitMask=bin2dec('100000000')  BitMaskRealWorld=Stored Integer
  Bitwise OR9 : simulink/Logic and Bit Operations/Bitwise Operator  logicop=AND  UseBitMask=on  BitMask=bin2dec('1000000000')  BitMaskRealWorld=Stored Integer
  Cast To Boolean{,1..15} (16 alike) : DataTypeConversion  OutDataTypeStr=boolean  SaturateOnIntegerOverflow=off  RndMeth=Floor
  Out1 : Outport  OutDataTypeStr=boolean
  Out2 : Outport  Port=2  OutDataTypeStr=boolean
  Out3 : Outport  Port=3  OutDataTypeStr=boolean
  Out4 : Outport  Port=4  OutDataTypeStr=boolean
  Out5 : Outport  Port=5  OutDataTypeStr=boolean
  Out6 : Outport  Port=6  OutDataTypeStr=boolean
  Out7 : Outport  Port=7  OutDataTypeStr=boolean
  Out8 : Outport  Port=8  OutDataTypeStr=boolean
  Out9 : Outport  Port=9  OutDataTypeStr=boolean
  Out10 : Outport  Port=10  OutDataTypeStr=boolean
  Out11 : Outport  Port=11  OutDataTypeStr=boolean
  Out12 : Outport  Port=12  OutDataTypeStr=boolean
  Out13 : Outport  Port=13  OutDataTypeStr=boolean
  Out14 : Outport  Port=14  OutDataTypeStr=boolean
  Out15 : Outport  Port=15  OutDataTypeStr=boolean
  Out16 : Outport  Port=16  OutDataTypeStr=boolean
  wires:
  Bitwise OR4/1 -> Cast To Boolean4/1
  Cast To Boolean2/1 -> Out3/1  "X"
  Bitwise OR2/1 -> Cast To Boolean2/1
  Bitwise OR5/1 -> Cast To Boolean5/1
  Cast To Boolean/1 -> Out1/1  "A"
  Bitwise OR9/1 -> Cast To Boolean9/1
  Input/1 -> Bitwise OR3/1, Bitwise OR15/1, Bitwise OR14/1, Bitwise OR13/1, Bitwise OR12/1, Bitwise OR11/1, Bitwise OR10/1, Bitwise OR9/1, Bitwise OR8/1, Bitwise OR7/1, Bitwise OR6/1, Bitwise OR5/1, Bitwise OR4/1, Bitwise OR2/1, Bitwise OR1/1, Bitwise OR/1  "ButtonBitField"
  Bitwise OR13/1 -> Cast To Boolean13/1
  Bitwise OR11/1 -> Cast To Boolean11/1
  Bitwise OR12/1 -> Cast To Boolean12/1
  Bitwise OR7/1 -> Cast To Boolean7/1
  Bitwise OR15/1 -> Cast To Boolean15/1
  Bitwise OR10/1 -> Cast To Boolean10/1
  Bitwise OR/1 -> Cast To Boolean/1
  Bitwise OR14/1 -> Cast To Boolean14/1
  Bitwise OR3/1 -> Cast To Boolean3/1
  Bitwise OR1/1 -> Cast To Boolean1/1
  Bitwise OR8/1 -> Cast To Boolean8/1
  Bitwise OR6/1 -> Cast To Boolean6/1
  Cast To Boolean1/1 -> Out2/1  "B"
  Cast To Boolean3/1 -> Out4/1  "Y"
  Cast To Boolean4/1 -> Out5/1  "LB"
  Cast To Boolean5/1 -> Out6/1  "RB"
  Cast To Boolean6/1 -> Out7/1  "LT"
  Cast To Boolean7/1 -> Out8/1  "RT"
  Cast To Boolean8/1 -> Out9/1  "BACK"
  Cast To Boolean9/1 -> Out10/1  "START"
  Cast To Boolean10/1 -> Out11/1  "LS"
  Cast To Boolean11/1 -> Out12/1  "RS"
  Cast To Boolean12/1 -> Out13/1  "UP"
  Cast To Boolean13/1 -> Out14/1  "DOWN"
  Cast To Boolean14/1 -> Out15/1  "LEFT"
  Cast To Boolean15/1 -> Out16/1  "RIGHT"

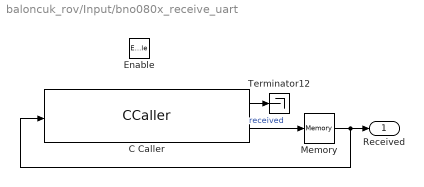
== system baloncuk_rov/Input/bno080x_receive_uart ==
  Enable : EnablePort
  C Caller : CCaller  FunctionName=bno08x_rvc_usart2_hal  PortSpecificationStruct="%)30     .    T ,   8    (     @         %    \"     (    !     0         %  0 \"0    $    _    07)G3F%M90  4&]R=$YA;64 4V-O<&4     26YD97@     5'EP90      4VEZ90      27-';&]B86P   X    P    !@    @    $          4    (     0    ,    !         !   P!O=70 #@   #     &    \"     0         !0    @    !     P    $         $  # &]U=  .    .     8    (    !          %    \"     $    &     0         0    !@   $]U='!U=   #@   #@    &    \"     8         !0    @    !     0    $         \"0    @               X    X    !@    @    $          4    (     0    <    !         !     '    8F]O;&5A;@ .    ,     8    (    !          %    \"     $    !     0         0  $ ,0    X    P    !@    @    ) @        4    (     0    $    !          (  0      #@   #@    &    \"     0         !0    @    !    \"     $         $     @   !R96-E:79E9 X    X    !@    @    $          4    (     0    @    !         !     (    <F5C96EV960.    0     8    (    !          %    \"     $    +     0         0    \"P   $EN<'5T3W5T<'5T       .    .     8    (    !@         %    \"     $    !     0         )    \"               #@   #@    &    \"     0         !0    @    !    !0    $         $     4   !U:6YT.     X    P    !@    @    $          4    (     0    (    !         !   @ Q.0  #@   #     &    \"     D\"        !0    @    !     0    $          @ !"
  Memory : Memory  InitialCondition=[uint8(0) uint8(0) uint8(0) uint8(0) uint8(0) uint8(0) uint8(0) uint8(0) uint8(0) uint8(0) uint8(0) uint8(0) uint8(0) uint8(0) uint8(0) uint8(0) uint8(0) uint8(0) uint8(0) ]
  Terminator12 : Terminator
  Received : Outport
  wires:
  C Caller/1 -> Terminator12/1
  C Caller/2 -> Memory/1  "received"
  Memory/1 -> Received/1, C Caller/1

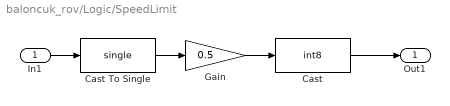
== system baloncuk_rov/Logic/SpeedLimit ==
  In1 : Inport
  Cast : DataTypeConversion  OutDataTypeStr=int8  SaturateOnIntegerOverflow=off  RndMeth=Floor
  Cast To Single : DataTypeConversion  OutDataTypeStr=single  SaturateOnIntegerOverflow=off  RndMeth=Floor
  Gain : Gain  Gain=0.5
  Out1 : Outport
  wires:
  In1/1 -> Cast To Single/1
  Cast To Single/1 -> Gain/1
  Gain/1 -> Cast/1
  Cast/1 -> Out1/1

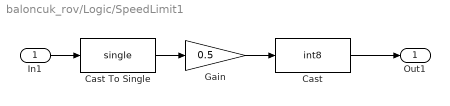
== system baloncuk_rov/Logic/SpeedLimit1 ==
  In1 : Inport
  Cast : DataTypeConversion  OutDataTypeStr=int8  SaturateOnIntegerOverflow=off  RndMeth=Floor
  Cast To Single : DataTypeConversion  OutDataTypeStr=single  SaturateOnIntegerOverflow=off  RndMeth=Floor
  Gain : Gain  Gain=0.5
  Out1 : Outport
  wires:
  Cast/1 -> Out1/1
  Gain/1 -> Cast/1
  Cast To Single/1 -> Gain/1
  In1/1 -> Cast To Single/1

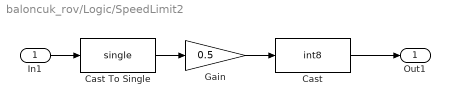
== system baloncuk_rov/Logic/SpeedLimit2 ==
  In1 : Inport
  Cast : DataTypeConversion  OutDataTypeStr=int8  SaturateOnIntegerOverflow=off  RndMeth=Floor
  Cast To Single : DataTypeConversion  OutDataTypeStr=single  SaturateOnIntegerOverflow=off  RndMeth=Floor
  Gain : Gain  Gain=0.5
  Out1 : Outport
  wires:
  In1/1 -> Cast To Single/1
  Cast To Single/1 -> Gain/1
  Gain/1 -> Cast/1
  Cast/1 -> Out1/1

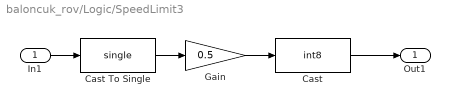
== system baloncuk_rov/Logic/SpeedLimit3 ==
  In1 : Inport
  Cast : DataTypeConversion  OutDataTypeStr=int8  SaturateOnIntegerOverflow=off  RndMeth=Floor
  Cast To Single : DataTypeConversion  OutDataTypeStr=single  SaturateOnIntegerOverflow=off  RndMeth=Floor
  Gain : Gain  Gain=0.5
  Out1 : Outport
  wires:
  Cast/1 -> Out1/1
  Gain/1 -> Cast/1
  Cast To Single/1 -> Gain/1
  In1/1 -> Cast To Single/1

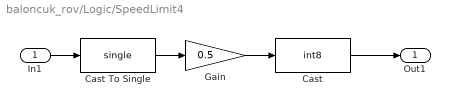
== system baloncuk_rov/Logic/SpeedLimit4 ==
  In1 : Inport
  Cast : DataTypeConversion  OutDataTypeStr=int8  SaturateOnIntegerOverflow=off  RndMeth=Floor
  Cast To Single : DataTypeConversion  OutDataTypeStr=single  SaturateOnIntegerOverflow=off  RndMeth=Floor
  Gain : Gain  Gain=0.5
  Out1 : Outport
  wires:
  In1/1 -> Cast To Single/1
  Cast To Single/1 -> Gain/1
  Gain/1 -> Cast/1
  Cast/1 -> Out1/1

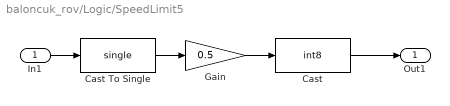
== system baloncuk_rov/Logic/SpeedLimit5 ==
  In1 : Inport
  Cast : DataTypeConversion  OutDataTypeStr=int8  SaturateOnIntegerOverflow=off  RndMeth=Floor
  Cast To Single : DataTypeConversion  OutDataTypeStr=single  SaturateOnIntegerOverflow=off  RndMeth=Floor
  Gain : Gain  Gain=0.5
  Out1 : Outport
  wires:
  Cast/1 -> Out1/1
  Gain/1 -> Cast/1
  Cast To Single/1 -> Gain/1
  In1/1 -> Cast To Single/1

== system baloncuk_rov/Output/Send_IMU_UDP_Enabled ==
  Data : Inport
  Enable : EnablePort
  Udp Send : stm32blockslib/Udp Send  Direction=Send  RemoteIPAddress=255.255.255.255  LocalPort=25011  RemoteIPPort=25011  ByteOrder=LittleEndian  BlockingMode=on  BlockTimeout=0.1  DataType=uint8  DataLength=1  OutputStatus=off
  wires:
  Data/1 -> Udp Send/1
